simulink model "Logic"  (R2025b)
settings: configuration reference "MCConfiguration" (kept outside this file)
settings Model: DataDictionary=embeddedBoard_common.sldd  Creator=rpumpo  LastModifiedBy=rpumpo
settings ConfigSetRef: SourceName=MCConfiguration

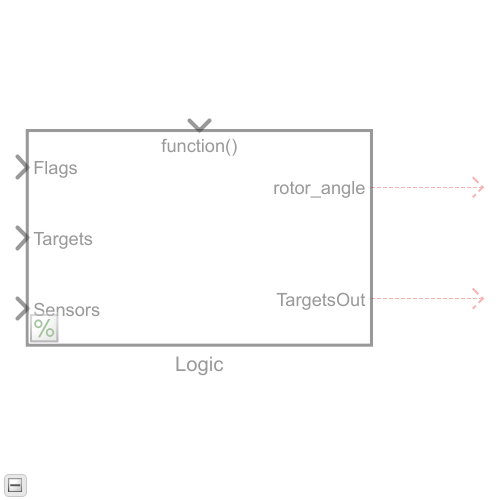
[thumbnail: Simulink's stored preview of the top-level diagram]
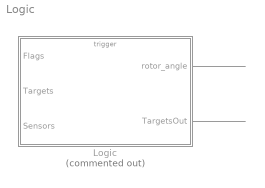
== system Logic ==
  Logic : Subsystem  Commented=on  TreatAsAtomicUnit=on
  wires:
  Logic/2(TargetsOut) -> ?
  Logic/1(rotor_angle) -> ?

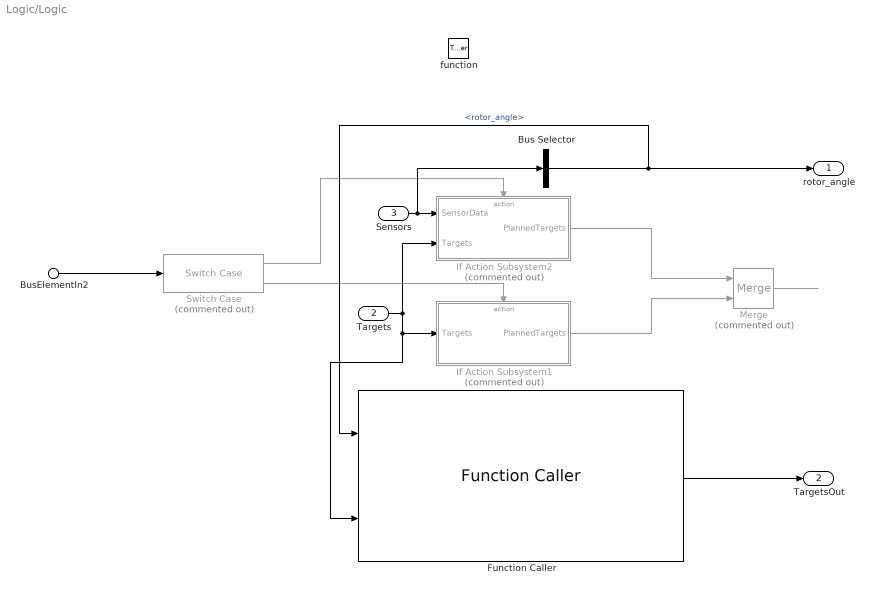
== system Logic/Logic ==
  BusElementIn2 : Inport  Description=control mode  PortName=Flags  Element=control_mode
  Targets : Inport  Port=2  OutDataTypeStr=Bus: Targets  BusOutputAsStruct=on
  Sensors : Inport  Port=3  OutDataTypeStr=Bus: SensorsData  BusOutputAsStruct=on
  function : TriggerPort  TriggerType=function-call  VariantControl=(inherit)
  Bus Selector : BusSelector  OutputSignals=motorsensors.qencoder.rotor_angle
  Function Caller : FunctionCaller  FunctionPrototype=planned_Targets = Planner.MinimumJerk(rotor_angle,Targets)  InputArgumentSpecifications=<Enter example>  OutputArgumentSpecifications=Targets
  If Action Subsystem1 : Subsystem  Commented=on  TreatAsAtomicUnit=on
  If Action Subsystem2 : Subsystem  Commented=on  TreatAsAtomicUnit=on
  Merge : Merge  Commented=on
  Switch Case : SwitchCase  Commented=on  CaseConditions={ControlModes.Position}
  rotor_angle : Outport
  TargetsOut : Outport  Port=2  OutDataTypeStr=Bus: Targets  BusOutputAsStruct=on
  wires:
  If Action Subsystem2/1(PlannedTargets) -> Merge/1
  If Action Subsystem1/1(PlannedTargets) -> Merge/2
  Switch Case/2 -> If Action Subsystem1/Action
  Merge/1 -> ?
  Switch Case/1 -> If Action Subsystem2/Action
  BusElementIn2/1 -> Switch Case/1
  Bus Selector/1 -> Function Caller/1, rotor_angle/1  "<rotor_angle>"
  Sensors/1 -> Bus Selector/1, If Action Subsystem2/1(SensorData)
  Targets/1 -> If Action Subsystem2/2(Targets), Function Caller/2, If Action Subsystem1/1(Targets)
  Function Caller/1 -> TargetsOut/1

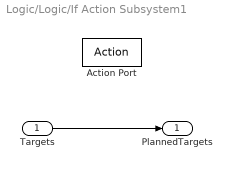
== system Logic/Logic/If Action Subsystem1 ==
  Targets : Inport  OutDataTypeStr=Bus: Targets
  Action Port : ActionPort  ActionPortLabel=default:
  PlannedTargets : Outport
  wires:
  Targets/1 -> PlannedTargets/1

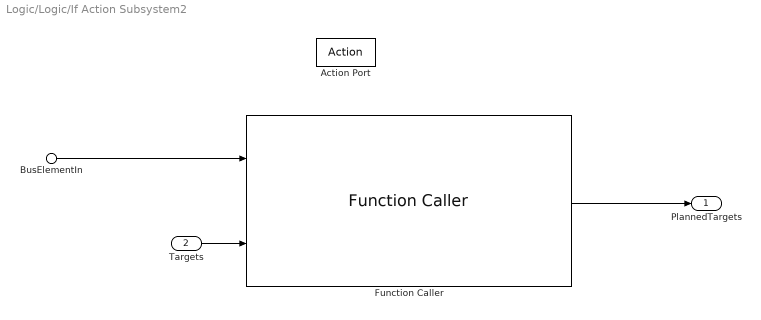
== system Logic/Logic/If Action Subsystem2 ==
  BusElementIn : Inport  Description=Mechanical Angle before gearbox  PortName=SensorData  Element=motorsensors.qencoder.rotor_angle
  Targets : Inport  Port=2  OutDataTypeStr=Bus: Targets
  Action Port : ActionPort  ActionPortLabel=case [ Position ]:
  Function Caller : FunctionCaller  FunctionPrototype=planned_Targets = Planner.MinimumJerk(rotor_angle,Targets)  InputArgumentSpecifications=<Enter example>  OutputArgumentSpecifications=Targets
  PlannedTargets : Outport  OutDataTypeStr=Bus: Targets
  wires:
  Targets/1 -> Function Caller/2
  Function Caller/1 -> PlannedTargets/1
  BusElementIn/1 -> Function Caller/1
